simulink model "PFC_V1_DRAFT"  (R2016b)
settings: Solver=FixedStepDiscrete  StartTime=0.0  StopTime=0.1  FixedStep=.1e-6  RelTol=1e-3
libraries: powerlib x41, simulink x4
settings Model: Creator=a037702  LastModifiedBy=a037702

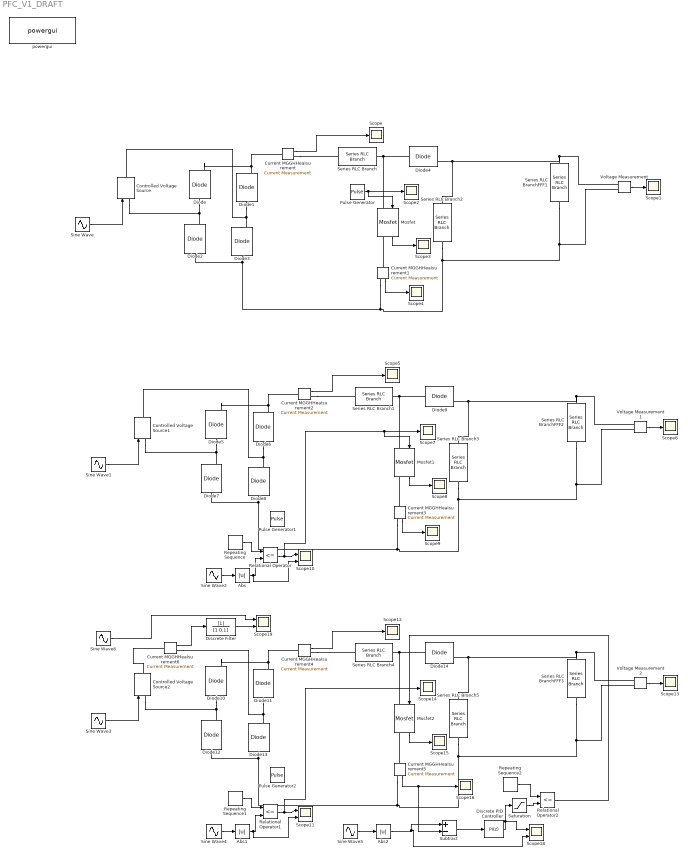
== system PFC_V1_DRAFT ==
  Abs : Abs
  Abs1 : Abs
  Abs2 : Abs
  Controlled Voltage Source : powerlib/Electrical Sources/Controlled Voltage Source  Initialize=on  Source_Type=AC  Amplitude=0  Phase=0  Frequency=0  Measurements=None
  Controlled Voltage Source1 : powerlib/Electrical Sources/Controlled Voltage Source  Initialize=on  Source_Type=AC  Amplitude=0  Phase=0  Frequency=0  Measurements=None
  Controlled Voltage Source2 : powerlib/Electrical Sources/Controlled Voltage Source  Initialize=on  Source_Type=AC  Amplitude=0  Phase=0  Frequency=0  Measurements=None
  Current MGGHHeaIsurement{,1..6} (7 alike) : powerlib/Measurements/Current Measurement  PhasorSimulation=off  OutputType=Complex  PSBequivalent=0
  Diode{,1..14} (15 alike) : powerlib/Power Electronics/Diode  Ron=0.001  Lon=0  Vf=0.8  IC=0  UseSnubber=off  Rs=500  Cs=250e-9  Measurements=on
  Discrete Filter : DiscreteFilter  Denominator=[1 0.1]
  Discrete PID Controller : simulink/Continuous/PID Controller  Controller=PI  TimeDomain=Discrete-time  SampleTime=-1  IntegratorMethod=Forward Euler  FilterMethod=Forward Euler  Form=Parallel  UseFilter=on  ControllerParametersSource=internal  P=0.001  I=100  D=0  N=100  InitialConditionSource=internal  InitialConditionForIntegrator=0  InitialConditionForFilter=0  ExternalReset=none  LimitOutput=off  UpperSaturationLimit=inf  LowerSaturationLimit=-inf  LinearizeAsGain=off  AntiWindupMode=none  Kb=1  TrackingMode=off  Kt=1  PParamMin=[]  PParamMax=[]  IParamMin=[]  IParamMax=[]  DParamMin=[]  DParamMax=[]  NParamMin=[]  NParamMax=[]  KbParamMin=[]  KbParamMax=[]  KtParamMin=[]  KtParamMax=[]  POutMin=[]  POutMax=[]  IOutMin=[]  IOutMax=[]  DOutMin=[]  DOutMax=[]  NOutMin=[]  NOutMax=[]  KbOutMin=[]  KbOutMax=[]  KtOutMin=[]  KtOutMax=[]  IntegratorOutMin=[]  IntegratorOutMax=[]  FilterOutMin=[]  FilterOutMax=[]  SumOutMin=[]  SumOutMax=[]  SumI1OutMin=[]  SumI1OutMax=[]  SumI2OutMin=[]  SumI2OutMax=[]  SumI3OutMin=[]  SumI3OutMax=[]  SumDOutMin=[]  SumDOutMax=[]  SaturationOutMin=[]  SaturationOutMax=[]  IntegratorContinuousStateAttributes=''  IntegratorStateMustResolveToSignalObject=off  IntegratorRTWStateStorageClass=Auto  FilterContinuousStateAttributes=''  FilterStateMustResolveToSignalObject=off  FilterRTWStateStorageClass=Auto  DifferentiatorICPrevScaledInput=0  DifferentiatorOutMin=[]  DifferentiatorOutMax=[]
  Mosfet : powerlib/Power Electronics/Mosfet  Ron=0.1  Lon=0  Rd=0.01  Vfd=0  IC=0  Rs=1e5  Cs=inf  Measurements=on
  Mosfet1 : powerlib/Power Electronics/Mosfet  Ron=0.1  Lon=0  Rd=0.01  Vfd=0  IC=0  Rs=1e5  Cs=inf  Measurements=on
  Mosfet2 : powerlib/Power Electronics/Mosfet  Ron=0.1  Lon=0  Rd=0.01  Vfd=0  IC=0  Rs=1e5  Cs=inf  Measurements=on
  Pulse Generator : DiscretePulseGenerator  PulseType=Time based  Amplitude=10  Period=10e-6  PulseWidth=50
  Pulse Generator1 : DiscretePulseGenerator  PulseType=Time based  Amplitude=10  Period=10e-6  PulseWidth=50
  Pulse Generator2 : DiscretePulseGenerator  PulseType=Time based  Amplitude=10  Period=10e-6  PulseWidth=50
  Relational Operator : RelationalOperator  Operator=<=  OutDataTypeStr=boolean  RndMeth=Simplest
  Relational Operator1 : RelationalOperator  Operator=<=  OutDataTypeStr=boolean  RndMeth=Simplest
  Relational Operator2 : RelationalOperator  Operator=<=  OutDataTypeStr=boolean  RndMeth=Simplest
  Repeating Sequence : simulink/Sources/Repeating Sequence  rep_seq_t=[0 10e-6]  rep_seq_y=[0 1]
  Repeating Sequence1 : simulink/Sources/Repeating Sequence  rep_seq_t=[0 10e-6]  rep_seq_y=[0 1]
  Repeating Sequence2 : simulink/Sources/Repeating Sequence  rep_seq_t=[0 10e-6]  rep_seq_y=[0 1]
  Saturation : Saturate  UpperLimit=0.95  LowerLimit=0.05
  Scope{,1..9,12..16} (15 alike) : Scope
  Scope{10..11,18..19} (4 alike) : Scope  NumInputPorts=2
  Series RLC Branch : powerlib/Elements/Series RLC Branch  LConnTagsString=__new0  RConnTagsString=__new0  BranchType=L  Resistance=1  Inductance=500e-6  SetiL0=on  InitialCurrent=0  Capacitance=1e-6  Setx0=off  InitialVoltage=0  Measurements=Branch current
  Series RLC Branch1 : powerlib/Elements/Series RLC Branch  LConnTagsString=__new0  RConnTagsString=__new0  BranchType=L  Resistance=1  Inductance=500e-6  SetiL0=on  InitialCurrent=0  Capacitance=1e-6  Setx0=off  InitialVoltage=0  Measurements=Branch current
  Series RLC Branch2 : powerlib/Elements/Series RLC Branch  LConnTagsString=__new0  RConnTagsString=__new0  BranchType=R  Resistance=100  Inductance=500e-6  SetiL0=on  InitialCurrent=0  Capacitance=100e-6  Setx0=on  InitialVoltage=0  Measurements=Branch current
  Series RLC Branch3 : powerlib/Elements/Series RLC Branch  LConnTagsString=__new0  RConnTagsString=__new0  BranchType=R  Resistance=100  Inductance=500e-6  SetiL0=on  InitialCurrent=0  Capacitance=100e-6  Setx0=on  InitialVoltage=0  Measurements=Branch current
  Series RLC Branch4 : powerlib/Elements/Series RLC Branch  LConnTagsString=__new0  RConnTagsString=__new0  BranchType=L  Resistance=1  Inductance=500e-6  SetiL0=on  InitialCurrent=0  Capacitance=1e-6  Setx0=off  InitialVoltage=0  Measurements=Branch current
  Series RLC Branch5 : powerlib/Elements/Series RLC Branch  LConnTagsString=__new0  RConnTagsString=__new0  BranchType=R  Resistance=100  Inductance=500e-6  SetiL0=on  InitialCurrent=0  Capacitance=100e-6  Setx0=on  InitialVoltage=0  Measurements=Branch current
  Series RLC BranchFFF1 : powerlib/Elements/Series RLC Branch  LConnTagsString=__new0  RConnTagsString=__new0  BranchType=C  Resistance=1  Inductance=500e-6  SetiL0=on  InitialCurrent=0  Capacitance=100e-6  Setx0=on  InitialVoltage=0  Measurements=Branch current
  Series RLC BranchFFF2 : powerlib/Elements/Series RLC Branch  LConnTagsString=__new0  RConnTagsString=__new0  BranchType=C  Resistance=1  Inductance=500e-6  SetiL0=on  InitialCurrent=0  Capacitance=100e-6  Setx0=on  InitialVoltage=0  Measurements=Branch current
  Series RLC BranchFFF3 : powerlib/Elements/Series RLC Branch  LConnTagsString=__new0  RConnTagsString=__new0  BranchType=C  Resistance=1  Inductance=500e-6  SetiL0=on  InitialCurrent=0  Capacitance=100e-6  Setx0=on  InitialVoltage=0  Measurements=Branch current
  Sine Wave : Sin  Amplitude=320  Frequency=2*pi*50  SampleTime=0
  Sine Wave1 : Sin  Amplitude=320  Frequency=2*pi*50  SampleTime=0
  Sine Wave2 : Sin  Amplitude=0.5  Frequency=2*pi*50  SampleTime=0
  Sine Wave3 : Sin  Amplitude=320  Frequency=2*pi*50  SampleTime=0
  Sine Wave4 : Sin  Amplitude=0.5  Frequency=2*pi*50  SampleTime=0
  Sine Wave5 : Sin  Amplitude=10  Frequency=2*pi*50  SampleTime=0
  Sine Wave6 : Sin  Amplitude=20  Frequency=2*pi*50  SampleTime=0
  Subtract : Sum  Inputs=+-
  Voltage Measurement : powerlib/Measurements/Voltage Measurement  PhasorSimulation=off  OutputType=Complex  PSBequivalent=0
  Voltage Measurement1 : powerlib/Measurements/Voltage Measurement  PhasorSimulation=off  OutputType=Complex  PSBequivalent=0
  Voltage Measurement2 : powerlib/Measurements/Voltage Measurement  PhasorSimulation=off  OutputType=Complex  PSBequivalent=0
  powergui : powerlib/powergui  Priority=1  SimulationMode=Discrete  SolverType=Tustin/Backward Euler (TBE)  SampleTime=.1e-6  frequency=60  SPID=off  DisableSnubberDevices=off  DisableRonSwitches=off  DisableVfSwitches=off  SwTol=0  DisplayEquations=off  Interpol=off  ExternalGateDelay=off  methode=off  Ts=10  FunctionMessages=off  echomessages=off  HookPort=off  EnableUseOfTLC=off  x0status=blocks  frequencyindice=0  Pbase=100e6  ErrMax=1e-4  Iterations=50  UnitsV=kV  UnitsW=MW  buscounter=0  RestoreLinks=warning  ResistiveCurrentMeasurement=off  Frange=[0:2:500]  Ylog=off  Xlog=on  ShowGrid=off  save=off  variable=ZData  structure=0  ZoomFFT=off  StartTime=0.0  cycles=1  DisplayStyle=1  fundamental=60  FreqAxis=off  MaxFrequency=1000  frequencyindicesteady=1  RmsSteady=1  display=off
  wires:
  Sine Wave/1 -> Controlled Voltage Source/1
  Current MGGHHeaIsurement/1 -> Scope/1
  Voltage Measurement/1 -> Scope1/1
  Pulse Generator/1 -> Mosfet/1, Scope2/1
  Mosfet/1 -> Scope3/1
  Current MGGHHeaIsurement1/1 -> Scope4/1
  Sine Wave1/1 -> Controlled Voltage Source1/1
  Current MGGHHeaIsurement2/1 -> Scope5/1
  Voltage Measurement1/1 -> Scope6/1
  Relational Operator/1 -> Mosfet1/1, Scope7/1, Scope10/1
  Mosfet1/1 -> Scope8/1
  Current MGGHHeaIsurement3/1 -> Scope9/1
  Sine Wave2/1 -> Abs/1
  Repeating Sequence/1 -> Relational Operator/1
  Abs/1 -> Scope10/2, Relational Operator/2
  Sine Wave3/1 -> Controlled Voltage Source2/1
  Current MGGHHeaIsurement4/1 -> Scope12/1
  Voltage Measurement2/1 -> Scope13/1
  Relational Operator1/1 -> Scope14/1, Scope11/1
  Mosfet2/1 -> Scope15/1
  Current MGGHHeaIsurement5/1 -> Subtract/2, Scope16/1
  Sine Wave4/1 -> Abs1/1
  Repeating Sequence1/1 -> Relational Operator1/1
  Abs1/1 -> Scope11/2, Relational Operator1/2
  Sine Wave5/1 -> Abs2/1
  Subtract/1 -> Discrete PID Controller/1
  Discrete PID Controller/1 -> Scope18/1, Saturation/1
  Saturation/1 -> Relational Operator2/2
  Repeating Sequence2/1 -> Relational Operator2/1
  Relational Operator2/1 -> Mosfet2/1
  Abs2/1 -> Scope18/2, Subtract/1
  Current MGGHHeaIsurement6/1 -> Discrete Filter/1
  Discrete Filter/1 -> Scope19/2
  Sine Wave6/1 -> Scope19/1
  connections:
  Diode1/RConn1 -- Diode/RConn1 -- Current MGGHHeaIsurement/LConn1
  Diode1/LConn1 -- Controlled Voltage Source/RConn1 -- Diode3/RConn1
  Diode/LConn1 -- Controlled Voltage Source/LConn1 -- Diode2/RConn1
  Diode3/LConn1 -- Series RLC Branch2/RConn1 -- Voltage Measurement/LConn2 -- Series RLC BranchFFF1/RConn1 -- Current MGGHHeaIsurement1/RConn1 -- Diode2/LConn1
  Current MGGHHeaIsurement/RConn1 -- Series RLC Branch/LConn1
  Series RLC Branch/RConn1 -- Diode4/LConn1 -- Mosfet/LConn1
  Series RLC BranchFFF1/LConn1 -- Voltage Measurement/LConn1 -- Series RLC Branch2/LConn1 -- Diode4/RConn1
  Current MGGHHeaIsurement1/LConn1 -- Mosfet/RConn1
  Diode6/RConn1 -- Diode5/RConn1 -- Current MGGHHeaIsurement2/LConn1
  Diode6/LConn1 -- Controlled Voltage Source1/RConn1 -- Diode8/RConn1
  Diode5/LConn1 -- Controlled Voltage Source1/LConn1 -- Diode7/RConn1
  Diode8/LConn1 -- Series RLC Branch3/RConn1 -- Voltage Measurement1/LConn2 -- Series RLC BranchFFF2/RConn1 -- Current MGGHHeaIsurement3/RConn1 -- Diode7/LConn1
  Series RLC Branch1/RConn1 -- Diode9/LConn1 -- Mosfet1/LConn1
  Series RLC BranchFFF2/LConn1 -- Voltage Measurement1/LConn1 -- Series RLC Branch3/LConn1 -- Diode9/RConn1
  Current MGGHHeaIsurement2/RConn1 -- Series RLC Branch1/LConn1
  Current MGGHHeaIsurement3/LConn1 -- Mosfet1/RConn1
  Diode11/RConn1 -- Diode10/RConn1 -- Current MGGHHeaIsurement4/LConn1
  Diode11/LConn1 -- Current MGGHHeaIsurement6/RConn1 -- Diode13/RConn1
  Diode10/LConn1 -- Controlled Voltage Source2/LConn1 -- Diode12/RConn1
  Diode13/LConn1 -- Diode12/LConn1 -- Current MGGHHeaIsurement5/RConn1 -- Series RLC Branch5/RConn1 -- Voltage Measurement2/LConn2 -- Series RLC BranchFFF3/RConn1
  Series RLC Branch4/RConn1 -- Diode14/LConn1 -- Mosfet2/LConn1
  Series RLC BranchFFF3/LConn1 -- Voltage Measurement2/LConn1 -- Series RLC Branch5/LConn1 -- Diode14/RConn1
  Current MGGHHeaIsurement4/RConn1 -- Series RLC Branch4/LConn1
  Current MGGHHeaIsurement5/LConn1 -- Mosfet2/RConn1
  Current MGGHHeaIsurement6/LConn1 -- Controlled Voltage Source2/RConn1
